simulink model "Soundtest"  (R2021a)
settings: Solver=FixedStepAuto  StartTime=0.0  StopTime=90  RelTol=1e-3
undefined symbols (not defined in the file): fdesignblkfcn, gcbh
libraries: simulink x25, simulink_extras x14, hdlsllib x9, eeGeneralControl x5, dspvision x4, commrandsrc3 x4, commutil2 x1
(part 1 of 5)
settings Model: Creator=PS  LastModifiedBy=PS

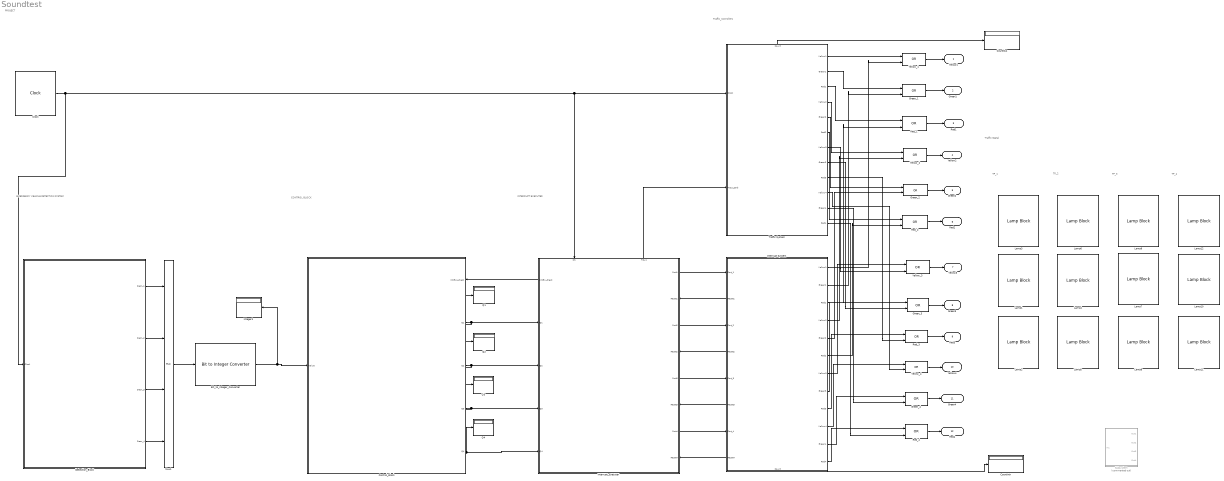
== system Soundtest ==
  note: INTERRUPT EXECUTER
  note: PROJECT
  note: CONTROL BLOCK
  note: EMERGENCY VEHICLE
      | 												DETECTION SYSTEM
  note: Traffic Signal
  note: Traffic_Conrollers
  note: TP_3
  note: TP_4
  note: TP_2
  note: TP_1
  " Control_Block" : Subsystem
      settings: PortSchema="{\"entries\":[{\"content\":{\"sides\":[{\"content\":{\"connectorIds\":[\"In1\"]},\"type\":\"ConnectorPlacement.EquallySpacedRectSide\",\"uuid\":\"7bdef495-49f6-4a33-afc1-3adee0384943\"},{\"content\":{\"connectorIds\":[\"In2\",\"Out1\",\"Out2\",\"Out3\",\"Out4\"],\"side\":\"RIGHT\"},\"type\":\"ConnectorPlacement.EquallySpacedRectSide\",\"uuid\":\"f7d0219f-f955-47d8-95dc-bc644c2b66ac\"},{\"content\":{\"connectorIds\":[],\"side\":\"TOP\"},\"type\":\"ConnectorPlacement.EquallySpacedRectSide\",\"uuid\":\"78ec8059-9416-4ba2-a7c7-38e9e6d506d5\"}]},\"type\":\"ConnectorPlacement.EquallySpacedConnector\",\"uuid\":\"6f2568f4-98e0-4465-825d-49049fff1cf4\"}],\"packageUris\":[\"http://schema.mathworks.com/mf0/Connector/R2020b\"],\"version\":\"1.0\"}"
  Bit_to_Integer_Converter : commutil2/Bit to Integer Converter  nbits=4  bitOrder=LSB first  signedOutputValues=Unsigned  outDtype=Inherit via internal rule  outDtypeSigned=Inherit via internal rule
  Clock : simulink_extras/Flip Flops/Clock  period=2
  CountIntr : Display
  CountSys : Display
  Detection_Block : Subsystem
  Green_{1..4} (4 alike) : Logic  Operator=OR  IconShape=distinctive  AllPortsSameDT=off  OutDataTypeStr=boolean
  Integer1 : Display
  Interrupt System : Subsystem
      settings: PortSchema="{\"entries\":[{\"content\":{\"sides\":[{\"content\":{\"connectorIds\":[\"In1\",\"Out14\",\"In2\",\"Out15\",\"In3\",\"Out16\",\"In4\",\"Out17\"]},\"type\":\"ConnectorPlacement.EquallySpacedRectSide\",\"uuid\":\"dd9361c9-50ac-49b9-98e3-b3d02327774e\"},{\"content\":{\"connectorIds\":[\"Out1\",\"Out2\",\"Out3\",\"Out4\",\"Out5\",\"Out6\",\"Out7\",\"Out8\",\"Out9\",\"Out10\",\"Out11\",\"Out12\"],\"side\":\"RIGHT\"},\"type\":\"ConnectorPlacement.EquallySpacedRectSide\",\"uuid\":\"f7e4faee-0171-4d20-8361-b22acdf13a20\"},{\"content\":{\"connectorIds\":[],\"side\":\"TOP\"},\"type\":\"ConnectorPlacement.EquallySpacedRectSide\",\"uuid\":\"5413f0d1-8ff5-4455-b45d-8db19df6353c\"},{\"content\":{\"connectorIds\":[\"Out13\"],\"side\":\"BOTTOM\"},\"type\":\"ConnectorPlacement.EquallySpacedRectSide\",\"uuid\":\"93b26c12-c259-4f39-b0b9-3af84b79bd60\"}]},\"type\":\"ConnectorPlacement.EquallySpacedConnector\",\"uuid\":\"eebdce44-6a00-4600-b51a-a6b58439fb08\"}],\"packageUris\":[\"http://schema.mathworks.com/mf0/Connector/R2020b\"],\"version\":\"1.0\"}"
  Interrupt_Executer : Subsystem
      settings: PortSchema="{\"entries\":[{\"content\":{\"sides\":[{\"content\":{\"connectorIds\":[\"Out6\",\"In1\",\"In2\",\"In3\",\"In4\"]},\"type\":\"ConnectorPlacement.EquallySpacedRectSide\",\"uuid\":\"f4bdf6e7-e5e7-43ea-b16b-e41e60f72b46\"},{\"content\":{\"connectorIds\":[\"Out1\",\"In6\",\"Out2\",\"In7\",\"Out3\",\"In8\",\"Out4\",\"In9\"],\"side\":\"RIGHT\"},\"type\":\"ConnectorPlacement.EquallySpacedRectSide\",\"uuid\":\"e5b218e6-0b4a-46b0-9989-01396b28dd8c\"},{\"content\":{\"connectorIds\":[\"In5\",\"Out5\"],\"side\":\"TOP\"},\"type\":\"ConnectorPlacement.EquallySpacedRectSide\",\"uuid\":\"ea6d06c9-d4c6-4cbd-a699-b09547b6713d\"}]},\"type\":\"ConnectorPlacement.EquallySpacedConnector\",\"uuid\":\"db6fa2d9-b0de-4c1a-aad1-7814046e63dd\"}],\"packageUris\":[\"http://schema.mathworks.com/mf0/Connector/R2020b\"],\"version\":\"1.0\"}"
  Lamp{1..12} (12 alike) : LampBlock
  Mux1 : Mux
  Q{1..4} (4 alike) : Display
  Red_{1..4} (4 alike) : Logic  Operator=OR  IconShape=distinctive  AllPortsSameDT=off  OutDataTypeStr=boolean
  Subsystem : Subsystem  Commented=on
  Traffic System : Subsystem
      settings: PortSchema="{\"entries\":[{\"content\":{\"sides\":[{\"content\":{\"connectorIds\":[\"In1\",\"In2\"]},\"type\":\"ConnectorPlacement.EquallySpacedRectSide\",\"uuid\":\"23d8ab70-c3d3-4b79-b104-f032a6dab7cf\"},{\"content\":{\"connectorIds\":[\"Out1\",\"Out2\",\"Out3\",\"Out4\",\"Out5\",\"Out6\",\"Out7\",\"Out8\",\"Out9\",\"Out10\",\"Out11\",\"Out12\"],\"side\":\"RIGHT\"},\"type\":\"ConnectorPlacement.EquallySpacedRectSide\",\"uuid\":\"7588026f-a2a4-4010-ad00-9eb40a03c993\"},{\"content\":{\"connectorIds\":[\"Out13\"],\"side\":\"TOP\"},\"type\":\"ConnectorPlacement.EquallySpacedRectSide\",\"uuid\":\"55eb16ed-4094-4229-af86-8dde9acd4f47\"}]},\"type\":\"ConnectorPlacement.EquallySpacedConnector\",\"uuid\":\"d987693c-4e87-4150-befb-2339b1a44195\"}],\"packageUris\":[\"http://schema.mathworks.com/mf0/Connector/R2020b\"],\"version\":\"1.0\"}"
  Yellow_{1..4} (4 alike) : Logic  Operator=OR  IconShape=distinctive  AllPortsSameDT=off  OutDataTypeStr=boolean
  Yellow1 : Outport  VectorParamsAs1DForOutWhenUnconnected=off
  Green1 : Outport  Port=2  VectorParamsAs1DForOutWhenUnconnected=off
  Red1 : Outport  Port=3  VectorParamsAs1DForOutWhenUnconnected=off
  Yellow2 : Outport  Port=4  VectorParamsAs1DForOutWhenUnconnected=off
  Green2 : Outport  Port=5  VectorParamsAs1DForOutWhenUnconnected=off
  Red2 : Outport  Port=6  VectorParamsAs1DForOutWhenUnconnected=off
  Yellow3 : Outport  Port=7  VectorParamsAs1DForOutWhenUnconnected=off
  Green3 : Outport  Port=8  VectorParamsAs1DForOutWhenUnconnected=off
  Red3 : Outport  Port=9  VectorParamsAs1DForOutWhenUnconnected=off
  Yellow4 : Outport  Port=10  VectorParamsAs1DForOutWhenUnconnected=off
  Green4 : Outport  Port=11  VectorParamsAs1DForOutWhenUnconnected=off
  Red4 : Outport  Port=12  VectorParamsAs1DForOutWhenUnconnected=off
  wires:
  Yellow_1/1 -> Yellow1/1
  Traffic System/1(Yellow1) -> Yellow_1/1
  Interrupt System/1(Yellow1) -> Yellow_1/2
  Traffic System/2(Green1) -> Green_1/1
  Interrupt System/2(Green1) -> Green_1/2
  Traffic System/3(Red1) -> Red_1/1
  Interrupt System/3(Red1) -> Red_1/2
  Traffic System/4(Yellow2) -> Yellow_2/1
  Interrupt System/4(Yellow2) -> Yellow_2/2
  Traffic System/5(Green2) -> Green_2/1
  Interrupt System/5(Green2) -> Green_2/2
  Green_1/1 -> Green1/1
  Red_1/1 -> Red1/1
  Yellow_2/1 -> Yellow2/1
  Green_2/1 -> Green2/1
  Traffic System/6(Red2) -> Red_2/1
  Interrupt System/6(Red2) -> Red_2/2
  Interrupt System/7(Yellow3) -> Yellow_3/1
  Traffic System/7(Yellow3) -> Yellow_3/2
  Traffic System/8(Green3) -> Green_3/2
  Interrupt System/8(Green3) -> Green_3/1
  Interrupt System/9(Red3) -> Red_3/1
  Traffic System/9(Red3) -> Red_3/2
  Interrupt System/10(Yellow4) -> Yellow_4/1
  Traffic System/10(Yellow4) -> Yellow_4/2
  Traffic System/11(Green4) -> Green_4/2
  Interrupt System/11(Green4) -> Green_4/1
  Interrupt System/12(Red4) -> Red_4/1
  Traffic System/12(Red4) -> Red_4/2
  Red_4/1 -> Red4/1
  Green_4/1 -> Green4/1
  Yellow_4/1 -> Yellow4/1
  Red_3/1 -> Red3/1
  Green_3/1 -> Green3/1
  Red_2/1 -> Red2/1
  Yellow_3/1 -> Yellow3/1
  Bit_to_Integer_Converter/1 -> Integer1/1, " Control_Block"/1(Value)
  Mux1/1 -> Bit_to_Integer_Converter/1
  Interrupt System/14(Reset1) -> Interrupt_Executer/6(Reset1)
  Interrupt System/15(Reset2) -> Interrupt_Executer/7(Reset2)
  Interrupt System/16(Reset3) -> Interrupt_Executer/8(Reset3)
  Interrupt System/17(Reset4) -> Interrupt_Executer/9(Reset4)
  Interrupt_Executer/5(TrSys) -> Traffic System/2(TrSys_Enb)
  Interrupt_Executer/6(IntrEx_check) -> " Control_Block"/2(IntrExc_check)
  Interrupt_Executer/1(Port1) -> Interrupt System/1(Port_1)
  Interrupt_Executer/2(Port2) -> Interrupt System/2(Port_2)
  Interrupt_Executer/3(Port3) -> Interrupt System/3(Port_3)
  Interrupt_Executer/4(Port4) -> Interrupt System/4(Port_4)
  " Control_Block"/1(Q1) -> Q1/1, Interrupt_Executer/1(Q1)
  " Control_Block"/2(Q2) -> Q2/1, Interrupt_Executer/2(Q2)
  " Control_Block"/3(Q3) -> Q3/1, Interrupt_Executer/3(Q3)
  " Control_Block"/4(Q4) -> Q4/1, Interrupt_Executer/4(Q4)
  Interrupt System/13(Count) -> CountIntr/1
  Traffic System/13(Count) -> CountSys/1
  Detection_Block/1(Decn_1) -> Mux1/1
  Detection_Block/2(Decn_2) -> Mux1/2
  Detection_Block/3(Decn_3) -> Mux1/3
  Detection_Block/4(Decn_4) -> Mux1/4
  Clock/1 -> Detection_Block/1(Clock), Traffic System/1(Clock), Interrupt_Executer/5(Clk)

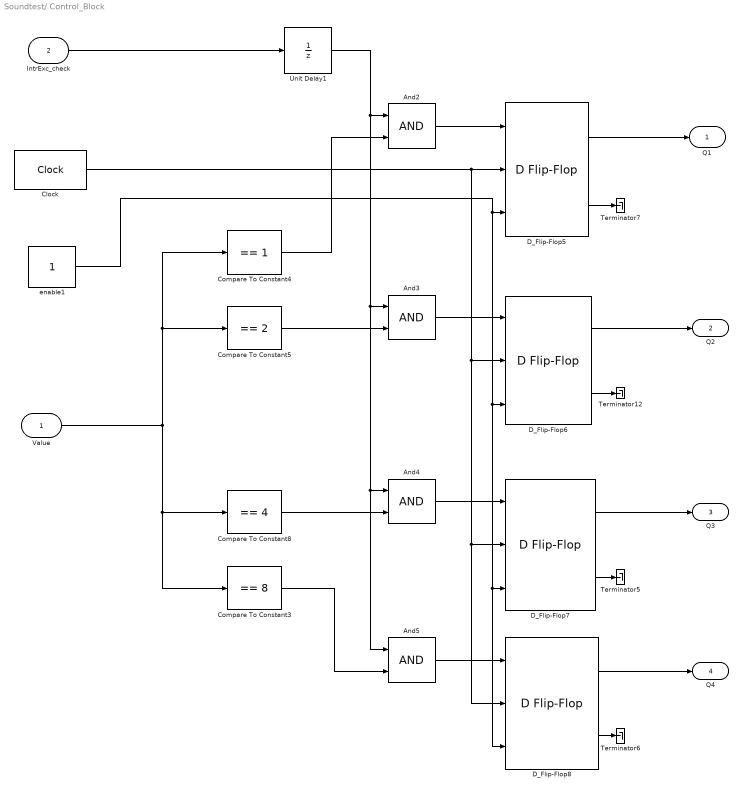
== system Soundtest/ Control_Block ==
  Value : Inport
  IntrExc_check : Inport  Port=2
  And{2..5} (4 alike) : Logic  IconShape=distinctive  AllPortsSameDT=off  OutDataTypeStr=boolean
  Clock : simulink_extras/Flip Flops/Clock  period=4
  Compare To Constant3 : simulink/Logic and Bit Operations/Compare To Constant  relop===  const=8  OutDataTypeStr=boolean
  Compare To Constant4 : simulink/Logic and Bit Operations/Compare To Constant  relop===  const=1  OutDataTypeStr=boolean
  Compare To Constant5 : simulink/Logic and Bit Operations/Compare To Constant  relop===  const=2  OutDataTypeStr=boolean
  Compare To Constant8 : simulink/Logic and Bit Operations/Compare To Constant  relop===  const=4  OutDataTypeStr=boolean
  D_Flip-Flop{5..8} (4 alike) : simulink_extras/Flip Flops/D Flip-Flop
  Terminator{5..7,12} (4 alike) : Terminator
  Unit Delay1 : UnitDelay  SampleTime=-1  HasFrameUpgradeWarning=on
  enable1 : Constant  OutDataTypeStr=boolean
  Q1 : Outport
  Q2 : Outport  Port=2
  Q3 : Outport  Port=3
  Q4 : Outport  Port=4
  wires:
  D_Flip-Flop8/1 -> Q4/1
  D_Flip-Flop5/1 -> Q1/1
  Clock/1 -> D_Flip-Flop5/2, D_Flip-Flop6/2, D_Flip-Flop7/2, D_Flip-Flop8/2
  enable1/1 -> D_Flip-Flop8/3, D_Flip-Flop7/3, D_Flip-Flop6/3, D_Flip-Flop5/3
  Compare To Constant5/1 -> And3/2
  Value/1 -> Compare To Constant4/1, Compare To Constant5/1, Compare To Constant3/1, Compare To Constant8/1
  And4/1 -> D_Flip-Flop7/1
  D_Flip-Flop6/2 -> Terminator12/1
  D_Flip-Flop6/1 -> Q2/1
  D_Flip-Flop7/1 -> Q3/1
  Compare To Constant8/1 -> And4/2
  D_Flip-Flop7/2 -> Terminator5/1
  D_Flip-Flop5/2 -> Terminator7/1
  And3/1 -> D_Flip-Flop6/1
  Unit Delay1/1 -> And2/1, And5/1, And4/1, And3/1
  Compare To Constant3/1 -> And5/2
  D_Flip-Flop8/2 -> Terminator6/1
  Compare To Constant4/1 -> And2/2
  And2/1 -> D_Flip-Flop5/1
  And5/1 -> D_Flip-Flop8/1
  IntrExc_check/1 -> Unit Delay1/1

== system Soundtest/Detection_Block ==
  Clock : Inport
  AND_{1..4} (4 alike) : Logic  IconShape=distinctive  AllPortsSameDT=off  OutDataTypeStr=boolean
  Ambulance_Detectors : Subsystem
  Constant : Constant  OutDataTypeStr=boolean
  D Flip-Flop1 : simulink_extras/Flip Flops/D Flip-Flop
  Enable : Constant  OutDataTypeStr=boolean
  Input_Sensors : Subsystem
  Scope : Scope  NumInputPorts=3
  Terminator2 : Terminator
  Decn_1 : Outport
  Decn_2 : Outport  Port=2
  Decn_3 : Outport  Port=3
  Decn_4 : Outport  Port=4
  wires:
  Input_Sensors/1(Inp_1) -> Ambulance_Detectors/1(Inp_1)
  Ambulance_Detectors/1(Filter_Out) -> Scope/1
  Input_Sensors/3(Inp_3) -> Ambulance_Detectors/3(Inp_3)
  Ambulance_Detectors/2(Mag_Out) -> Scope/2
  Input_Sensors/2(Inp_2) -> Ambulance_Detectors/2(Inp_2)
  Input_Sensors/4(Inp_4) -> Ambulance_Detectors/4(Inp_4)
  Ambulance_Detectors/3(Decn_1) -> AND_1/1, Scope/3
  Ambulance_Detectors/4(Decn_2) -> AND_2/1
  Constant/1 -> D Flip-Flop1/1
  D Flip-Flop1/2 -> Terminator2/1
  Enable/1 -> D Flip-Flop1/3
  Clock/1 -> D Flip-Flop1/2
  AND_2/1 -> Decn_2/1
  AND_3/1 -> Decn_3/1
  Ambulance_Detectors/5(Decn_3) -> AND_3/1
  Ambulance_Detectors/6(Decn_4) -> AND_4/1
  AND_4/1 -> Decn_4/1
  D Flip-Flop1/1 -> AND_1/2, AND_2/2, AND_3/2, AND_4/2
  AND_1/1 -> Decn_1/1

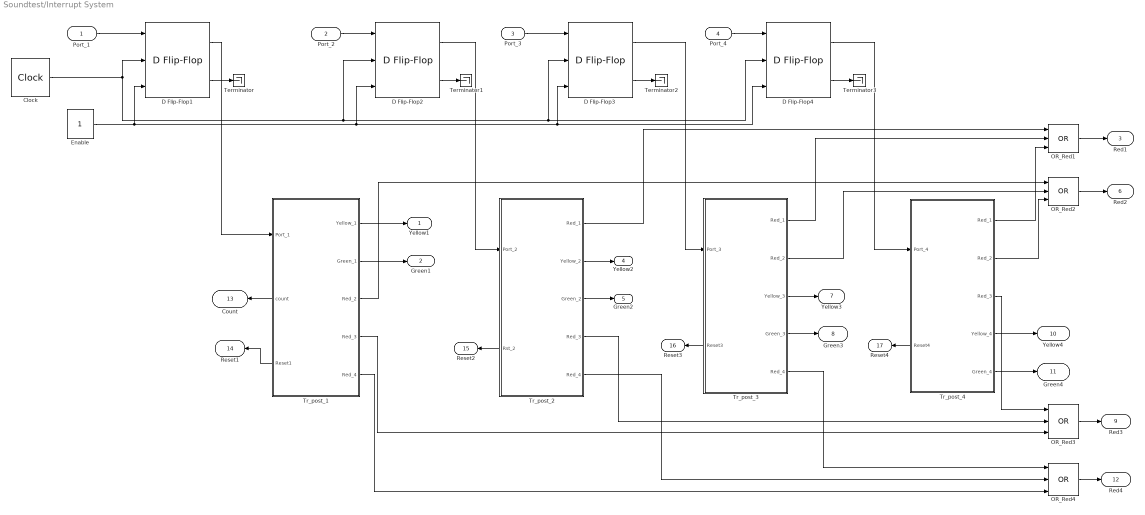
== system Soundtest/Interrupt System ==
  Port_1 : Inport
  Port_2 : Inport  Port=2
  Port_3 : Inport  Port=3
  Port_4 : Inport  Port=4
  Clock : simulink_extras/Flip Flops/Clock  period=2
  D Flip-Flop{1..4} (4 alike) : simulink_extras/Flip Flops/D Flip-Flop
  Enable : Constant  OutDataTypeStr=boolean
  OR_Red{1..4} (4 alike) : Logic  Operator=OR  Inputs=3  IconShape=distinctive  AllPortsSameDT=off  OutDataTypeStr=boolean
  Terminator{,1..3} (4 alike) : Terminator
  Tr_post_1 : Subsystem
      settings: PortSchema="{\"entries\":[{\"content\":{\"sides\":[{\"content\":{\"connectorIds\":[\"In1\",\"Out6\",\"Out7\"]},\"type\":\"ConnectorPlacement.EquallySpacedRectSide\",\"uuid\":\"ab8f469e-3332-475a-83d5-afbd6f66f4e6\"},{\"content\":{\"connectorIds\":[\"Out1\",\"Out2\",\"Out3\",\"Out4\",\"Out5\"],\"side\":\"RIGHT\"},\"type\":\"ConnectorPlacement.EquallySpacedRectSide\",\"uuid\":\"6823faed-dca4-4af2-a519-b6f8f71579c8\"},{\"content\":{\"connectorIds\":[],\"side\":\"TOP\"},\"type\":\"ConnectorPlacement.EquallySpacedRectSide\",\"uuid\":\"8d9facd3-edb6-42bc-be5d-0022a243b86f\"}]},\"type\":\"ConnectorPlacement.EquallySpacedConnector\",\"uuid\":\"a2e4fdf2-469e-412a-bc2f-0a5c51d0db72\"}],\"packageUris\":[\"http://schema.mathworks.com/mf0/Connector/R2020b\"],\"version\":\"1.0\"}"
  Tr_post_2 : Subsystem
      settings: PortSchema="{\"entries\":[{\"content\":{\"sides\":[{\"content\":{\"connectorIds\":[\"In1\",\"Out6\"]},\"type\":\"ConnectorPlacement.EquallySpacedRectSide\",\"uuid\":\"cf8efb98-dcb3-4b52-bb29-44068cf36b42\"},{\"content\":{\"connectorIds\":[\"Out1\",\"Out2\",\"Out3\",\"Out4\",\"Out5\"],\"side\":\"RIGHT\"},\"type\":\"ConnectorPlacement.EquallySpacedRectSide\",\"uuid\":\"3b505268-83a1-4950-b579-e5c30ad50a49\"},{\"content\":{\"connectorIds\":[],\"side\":\"TOP\"},\"type\":\"ConnectorPlacement.EquallySpacedRectSide\",\"uuid\":\"d6f0b650-deb9-4fd5-a2d1-5d40893a956e\"}]},\"type\":\"ConnectorPlacement.EquallySpacedConnector\",\"uuid\":\"7382f276-3b35-4664-8acb-0fe9e679eb95\"}],\"packageUris\":[\"http://schema.mathworks.com/mf0/Connector/R2020b\"],\"version\":\"1.0\"}"
  Tr_post_3 : Subsystem
      settings: PortSchema="{\"entries\":[{\"content\":{\"sides\":[{\"content\":{\"connectorIds\":[\"In1\",\"Out6\"]},\"type\":\"ConnectorPlacement.EquallySpacedRectSide\",\"uuid\":\"cf8efb98-dcb3-4b52-bb29-44068cf36b42\"},{\"content\":{\"connectorIds\":[\"Out1\",\"Out2\",\"Out3\",\"Out4\",\"Out5\"],\"side\":\"RIGHT\"},\"type\":\"ConnectorPlacement.EquallySpacedRectSide\",\"uuid\":\"3b505268-83a1-4950-b579-e5c30ad50a49\"},{\"content\":{\"connectorIds\":[],\"side\":\"TOP\"},\"type\":\"ConnectorPlacement.EquallySpacedRectSide\",\"uuid\":\"d6f0b650-deb9-4fd5-a2d1-5d40893a956e\"}]},\"type\":\"ConnectorPlacement.EquallySpacedConnector\",\"uuid\":\"7382f276-3b35-4664-8acb-0fe9e679eb95\"}],\"packageUris\":[\"http://schema.mathworks.com/mf0/Connector/R2020b\"],\"version\":\"1.0\"}"
  Tr_post_4 : Subsystem
      settings: PortSchema="{\"entries\":[{\"content\":{\"sides\":[{\"content\":{\"connectorIds\":[\"In1\",\"Out6\"]},\"type\":\"ConnectorPlacement.EquallySpacedRectSide\",\"uuid\":\"cf8efb98-dcb3-4b52-bb29-44068cf36b42\"},{\"content\":{\"connectorIds\":[\"Out1\",\"Out2\",\"Out3\",\"Out4\",\"Out5\"],\"side\":\"RIGHT\"},\"type\":\"ConnectorPlacement.EquallySpacedRectSide\",\"uuid\":\"3b505268-83a1-4950-b579-e5c30ad50a49\"},{\"content\":{\"connectorIds\":[],\"side\":\"TOP\"},\"type\":\"ConnectorPlacement.EquallySpacedRectSide\",\"uuid\":\"d6f0b650-deb9-4fd5-a2d1-5d40893a956e\"}]},\"type\":\"ConnectorPlacement.EquallySpacedConnector\",\"uuid\":\"7382f276-3b35-4664-8acb-0fe9e679eb95\"}],\"packageUris\":[\"http://schema.mathworks.com/mf0/Connector/R2020b\"],\"version\":\"1.0\"}"
  Yellow1 : Outport
  Green1 : Outport  Port=2
  Red1 : Outport  Port=3
  Yellow2 : Outport  Port=4
  Green2 : Outport  Port=5
  Red2 : Outport  Port=6
  Yellow3 : Outport  Port=7
  Green3 : Outport  Port=8
  Red3 : Outport  Port=9
  Yellow4 : Outport  Port=10
  Green4 : Outport  Port=11
  Red4 : Outport  Port=12
  Count : Outport  Port=13
  Reset1 : Outport  Port=14
  Reset2 : Outport  Port=15
  Reset3 : Outport  Port=16
  Reset4 : Outport  Port=17
  wires:
  Tr_post_2/2(Yellow_2) -> Yellow2/1
  Tr_post_3/3(Yellow_3) -> Yellow3/1
  Tr_post_3/4(Green_3) -> Green3/1
  Tr_post_4/5(Green_4) -> Green4/1
  Tr_post_4/4(Yellow_4) -> Yellow4/1
  Tr_post_2/3(Green_2) -> Green2/1
  OR_Red1/1 -> Red1/1
  Tr_post_1/2(Green_1) -> Green1/1
  Tr_post_1/1(Yellow_1) -> Yellow1/1
  OR_Red2/1 -> Red2/1
  OR_Red4/1 -> Red4/1
  OR_Red3/1 -> Red3/1
  Tr_post_2/1(Red_1) -> OR_Red1/1
  Tr_post_3/1(Red_1) -> OR_Red1/2
  Tr_post_4/1(Red_1) -> OR_Red1/3
  Tr_post_1/3(Red_2) -> OR_Red2/1
  Tr_post_3/2(Red_2) -> OR_Red2/2
  Tr_post_4/2(Red_2) -> OR_Red2/3
  Tr_post_1/4(Red_3) -> OR_Red3/3
  Tr_post_2/4(Red_3) -> OR_Red3/2
  Tr_post_4/3(Red_3) -> OR_Red3/1
  Tr_post_1/5(Red_4) -> OR_Red4/3
  Tr_post_2/5(Red_4) -> OR_Red4/2
  Tr_post_3/5(Red_4) -> OR_Red4/1
  Tr_post_1/7(Reset1) -> Reset1/1
  Tr_post_2/6(Rst_2) -> Reset2/1
  Tr_post_3/6(Reset3) -> Reset3/1
  Tr_post_4/6(Reset4) -> Reset4/1
  D Flip-Flop1/1 -> Tr_post_1/1(Port_1)
  Port_1/1 -> D Flip-Flop1/1
  D Flip-Flop1/2 -> Terminator/1
  D Flip-Flop2/1 -> Tr_post_2/1(Port_2)
  D Flip-Flop2/2 -> Terminator1/1
  Port_2/1 -> D Flip-Flop2/1
  D Flip-Flop3/1 -> Tr_post_3/1(Port_3)
  Port_3/1 -> D Flip-Flop3/1
  D Flip-Flop3/2 -> Terminator2/1
  Port_4/1 -> D Flip-Flop4/1
  D Flip-Flop4/2 -> Terminator3/1
  Clock/1 -> D Flip-Flop1/2, D Flip-Flop2/2, D Flip-Flop4/2, D Flip-Flop3/2
  Enable/1 -> D Flip-Flop4/3, D Flip-Flop3/3, D Flip-Flop2/3, D Flip-Flop1/3
  D Flip-Flop4/1 -> Tr_post_4/1(Port_4)
  Tr_post_1/6(count) -> Count/1

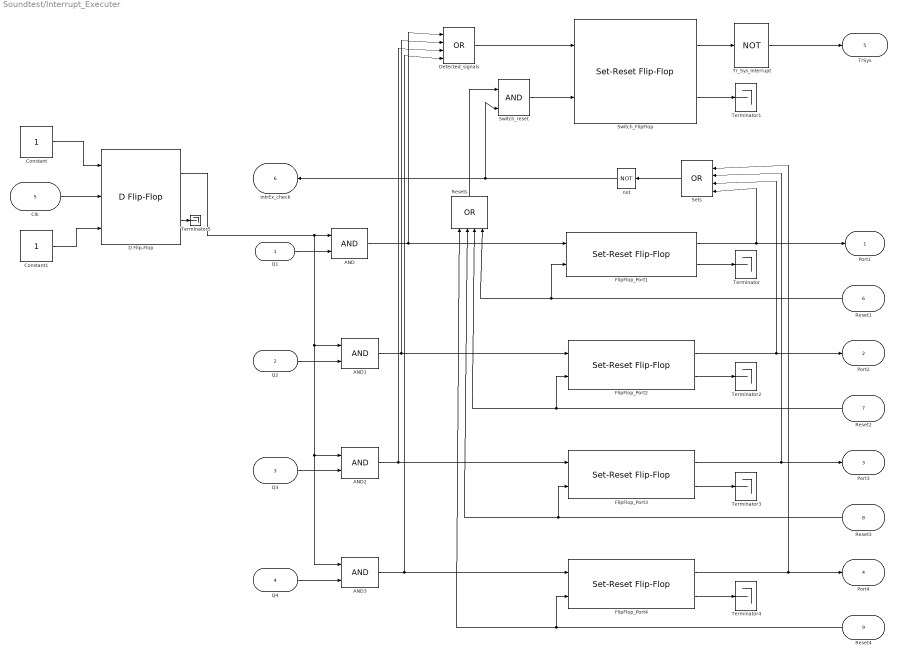
== system Soundtest/Interrupt_Executer ==
  Q1 : Inport
  Q2 : Inport  Port=2
  Q3 : Inport  Port=3
  Q4 : Inport  Port=4
  Clk : Inport  Port=5
  Reset1 : Inport  Port=6
  Reset2 : Inport  Port=7
  Reset3 : Inport  Port=8
  Reset4 : Inport  Port=9
  AND{,1..3} (4 alike) : Logic  IconShape=distinctive  AllPortsSameDT=off  OutDataTypeStr=boolean
  Constant : Constant  OutDataTypeStr=boolean
  Constant1 : Constant  OutDataTypeStr=boolean
  D Flip-Flop : simulink_extras/Flip Flops/D Flip-Flop
  Detected_signals : Logic  Operator=OR  Inputs=4  IconShape=distinctive  AllPortsSameDT=off  OutDataTypeStr=boolean
  FlipFlop_Port{1..4} (4 alike) : eeGeneralControl/Set-Reset Flip-Flop  LabelModeActiveChoice=Discrete  UndefState=Set  Q0=0  Ts=-1
      settings: SourceProductBaseCode=PS
  Resets : Logic  Operator=OR  Inputs=4  IconShape=distinctive  AllPortsSameDT=off  OutDataTypeStr=boolean
  Sets : Logic  Operator=OR  Inputs=4  IconShape=distinctive  AllPortsSameDT=off  OutDataTypeStr=boolean
  Switch_FlipFlop : eeGeneralControl/Set-Reset Flip-Flop  LabelModeActiveChoice=Discrete  UndefState=Set  Q0=0  Ts=-1
      settings: SourceProductBaseCode=PS
  Switch_reset : Logic  IconShape=distinctive  AllPortsSameDT=off  OutDataTypeStr=boolean
  Terminator{,1..5} (6 alike) : Terminator
  Tr_Sys_Interrupt : Logic  Operator=NOT  Inputs=4  IconShape=distinctive  AllPortsSameDT=off  OutDataTypeStr=boolean
  not : Logic  Operator=NOT  Inputs=4  IconShape=distinctive  AllPortsSameDT=off  OutDataTypeStr=boolean
  Port1 : Outport
  Port2 : Outport  Port=2
  Port3 : Outport  Port=3
  Port4 : Outport  Port=4
  TrSys : Outport  Port=5
  IntrEx_check : Outport  Port=6
  wires:
  FlipFlop_Port1/1 -> Sets/4, Port1/1
  Switch_reset/1 -> Switch_FlipFlop/2
  Reset2/1 -> FlipFlop_Port2/2, Resets/3
  FlipFlop_Port2/2 -> Terminator2/1
  Switch_FlipFlop/1 -> Tr_Sys_Interrupt/1
  FlipFlop_Port2/1 -> Sets/3, Port2/1
  AND1/1 -> Detected_signals/2, FlipFlop_Port2/1
  AND3/1 -> Detected_signals/4, FlipFlop_Port4/1
  Reset3/1 -> FlipFlop_Port3/2, Resets/2
  Switch_FlipFlop/2 -> Terminator1/1
  not/1 -> Switch_reset/2, IntrEx_check/1
  Reset1/1 -> Resets/4, FlipFlop_Port1/2
  Sets/1 -> not/1
  Resets/1 -> Switch_reset/1
  FlipFlop_Port3/2 -> Terminator3/1
  AND2/1 -> Detected_signals/3, FlipFlop_Port3/1
  FlipFlop_Port3/1 -> Sets/2, Port3/1
  Tr_Sys_Interrupt/1 -> TrSys/1
  FlipFlop_Port4/2 -> Terminator4/1
  Reset4/1 -> FlipFlop_Port4/2, Resets/1
  Detected_signals/1 -> Switch_FlipFlop/1
  FlipFlop_Port4/1 -> Sets/1, Port4/1
  FlipFlop_Port1/2 -> Terminator/1
  AND/1 -> Detected_signals/1, FlipFlop_Port1/1
  Constant/1 -> D Flip-Flop/1
  Clk/1 -> D Flip-Flop/2
  Constant1/1 -> D Flip-Flop/3
  Q1/1 -> AND/2
  D Flip-Flop/1 -> AND3/1, AND2/1, AND1/1, AND/1
  Q2/1 -> AND1/2
  Q3/1 -> AND2/2
  Q4/1 -> AND3/2
  D Flip-Flop/2 -> Terminator5/1

== system Soundtest/Subsystem ==
  note: Binary_Generator
  In1 : Inport
  AND{,1..3} (4 alike) : Logic  IconShape=distinctive  AllPortsSameDT=off  OutDataTypeStr=boolean
  Bernoulli Binary Generator : commrandsrc3/Bernoulli Binary Generator  ProbabilityOfZero=1  SeedSource=Auto  Seed=0  SampleTime=1  SamplesPerFrame=1  OutputDataType=boolean  SimulateUsing=Interpreted execution
  Bernoulli Binary Generator1 : commrandsrc3/Bernoulli Binary Generator  ProbabilityOfZero=0.8  SeedSource=Auto  Seed=0  SampleTime=1  SamplesPerFrame=1  OutputDataType=boolean  SimulateUsing=Interpreted execution
  Bernoulli Binary Generator2 : commrandsrc3/Bernoulli Binary Generator  ProbabilityOfZero=0.8  SeedSource=Auto  Seed=0  SampleTime=1  SamplesPerFrame=1  OutputDataType=boolean  SimulateUsing=Interpreted execution
  Bernoulli Binary Generator3 : commrandsrc3/Bernoulli Binary Generator  ProbabilityOfZero=0.8  SeedSource=Auto  Seed=0  SampleTime=1  SamplesPerFrame=1  OutputDataType=boolean  SimulateUsing=Interpreted execution
  Out1 : Outport
  Out2 : Outport  Port=2
  Out3 : Outport  Port=3
  Out4 : Outport  Port=4
  wires:
  Bernoulli Binary Generator/1 -> AND/1
  Bernoulli Binary Generator3/1 -> AND3/1
  Bernoulli Binary Generator2/1 -> AND2/1
  Bernoulli Binary Generator1/1 -> AND1/2
  In1/1 -> AND3/2, AND2/2, AND1/1, AND/2
  AND2/1 -> Out3/1
  AND3/1 -> Out4/1
  AND1/1 -> Out2/1
  AND/1 -> Out1/1

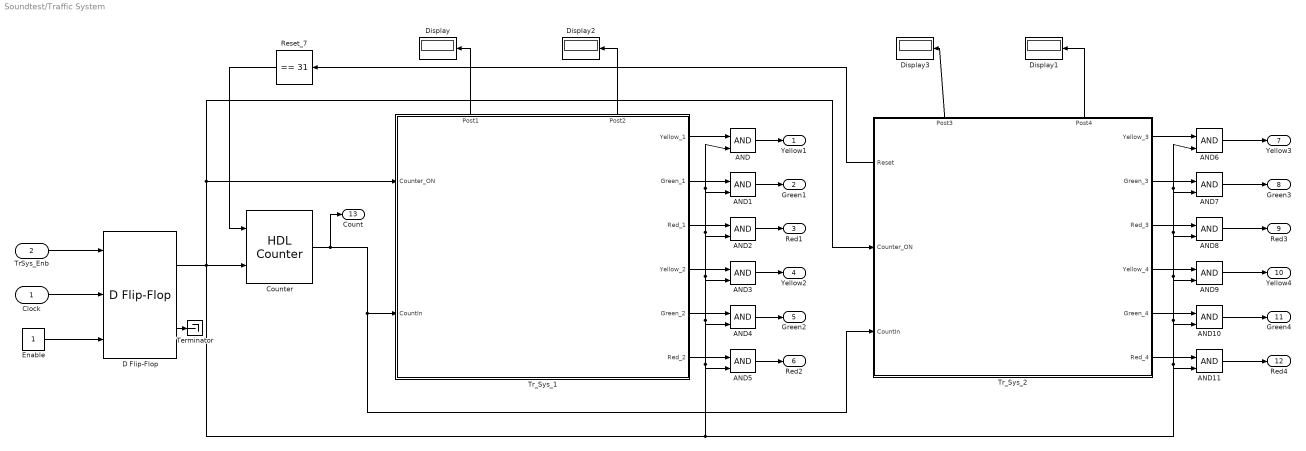
== system Soundtest/Traffic System ==
  Clock : Inport
  TrSys_Enb : Inport  Port=2
  AND{,1..11} (12 alike) : Logic  IconShape=distinctive  AllPortsSameDT=off  OutDataTypeStr=boolean
  Counter : hdlsllib/Sources/HDL Counter  CountType=Count limited  CountInit=0  CountStep=1  CountMax=31  CountFromType=Initial value  CountFrom=0  CountResetPort=on  CountLoadPort=off  CountEnbPort=on  CountDirPort=off  CountHitOutputPort=off  CountDataType=Unsigned  CountWordLen=8  CountFracLen=0  CountSampTime=1
  D Flip-Flop : simulink_extras/Flip Flops/D Flip-Flop
  Display{,1..3} (4 alike) : Display
  Enable : Constant  OutDataTypeStr=boolean
  Reset_7 : simulink/Logic and Bit Operations/Compare To Constant  relop===  const=31  OutDataTypeStr=boolean
  Terminator : Terminator
  Tr_Sys_1 : Subsystem
      settings: PortSchema="{\"entries\":[{\"content\":{\"sides\":[{\"content\":{\"connectorIds\":[\"In1\",\"In2\"]},\"type\":\"ConnectorPlacement.EquallySpacedRectSide\",\"uuid\":\"cd6a573a-f63a-4267-a232-9eb42b0e4457\"},{\"content\":{\"connectorIds\":[\"Out1\",\"Out2\",\"Out3\",\"Out4\",\"Out5\",\"Out6\"],\"side\":\"RIGHT\"},\"type\":\"ConnectorPlacement.EquallySpacedRectSide\",\"uuid\":\"f6eb4910-c6df-488e-ab3b-2d26710c7ea4\"},{\"content\":{\"connectorIds\":[\"Out7\",\"Out8\"],\"side\":\"TOP\"},\"type\":\"ConnectorPlacement.EquallySpacedRectSide\",\"uuid\":\"a673d499-f1f0-4298-be23-50c47df79d07\"}]},\"type\":\"ConnectorPlacement.EquallySpacedConnector\",\"uuid\":\"fa6e7a6f-15f6-4fb6-9f68-54e163a559b7\"}],\"packageUris\":[\"http://schema.mathworks.com/mf0/Connector/R2020b\"],\"version\":\"1.0\"}"
  Tr_Sys_2 : Subsystem
      settings: PortSchema="{\"entries\":[{\"content\":{\"sides\":[{\"content\":{\"connectorIds\":[\"Out9\",\"In1\",\"In2\"]},\"type\":\"ConnectorPlacement.EquallySpacedRectSide\",\"uuid\":\"f688e7f2-a4b0-4876-aa54-3ea0bbaacfd9\"},{\"content\":{\"connectorIds\":[\"Out1\",\"Out2\",\"Out3\",\"Out4\",\"Out5\",\"Out6\"],\"side\":\"RIGHT\"},\"type\":\"ConnectorPlacement.EquallySpacedRectSide\",\"uuid\":\"7fe066cd-bdaf-47f1-a6ea-f29d6eb723dd\"},{\"content\":{\"connectorIds\":[\"Out7\",\"Out8\"],\"side\":\"TOP\"},\"type\":\"ConnectorPlacement.EquallySpacedRectSide\",\"uuid\":\"39c29f91-5efa-4dbe-99ee-6bedb48eb38c\"},{\"content\":{\"connectorIds\":[],\"side\":\"BOTTOM\"},\"type\":\"ConnectorPlacement.EquallySpacedRectSide\",\"uuid\":\"136e34fe-1c95-412d-a8c7-b895a3917e8c\"}]},\"type\":\"ConnectorPlacement.EquallySpacedConnector\",\"uuid\":\"b68eec12-5eae-464b-ad0d-c0eefae3b870\"}],\"packageUris\":[\"http://schema.mathworks.com/mf0/Connector/R2020b\"],\"version\":\"1.0\"}"
  Yellow1 : Outport
  Green1 : Outport  Port=2
  Red1 : Outport  Port=3
  Yellow2 : Outport  Port=4
  Green2 : Outport  Port=5
  Red2 : Outport  Port=6
  Yellow3 : Outport  Port=7
  Green3 : Outport  Port=8
  Red3 : Outport  Port=9
  Yellow4 : Outport  Port=10
  Green4 : Outport  Port=11
  Red4 : Outport  Port=12
  Count : Outport  Port=13
  wires:
  Tr_Sys_2/9(Reset) -> Reset_7/1
  Reset_7/1 -> Counter/1
  D Flip-Flop/1 -> AND11/2, AND9/2, AND8/2, AND7/2, AND6/2, AND10/2, AND5/2, AND4/2, AND3/2, AND2/2, AND1/2, AND/2, Tr_Sys_1/1(Counter_ON), Tr_Sys_2/1(Counter_ON), Counter/2
  Tr_Sys_1/1(Yellow_1) -> AND/1
  AND/1 -> Yellow1/1
  Tr_Sys_1/2(Green_1) -> AND1/1
  AND4/1 -> Green2/1
  AND5/1 -> Red2/1
  AND3/1 -> Yellow2/1
  AND2/1 -> Red1/1
  AND1/1 -> Green1/1
  AND6/1 -> Yellow3/1
  Tr_Sys_2/6(Red_4) -> AND11/1
  Tr_Sys_2/5(Green_4) -> AND10/1
  Tr_Sys_2/4(Yellow_4) -> AND9/1
  Tr_Sys_2/3(Red_3) -> AND8/1
  Tr_Sys_2/2(Green_3) -> AND7/1
  Tr_Sys_2/1(Yellow_3) -> AND6/1
  AND11/1 -> Red4/1
  AND10/1 -> Green4/1
  AND9/1 -> Yellow4/1
  AND8/1 -> Red3/1
  AND7/1 -> Green3/1
  Tr_Sys_1/5(Green_2) -> AND4/1
  Tr_Sys_1/6(Red_2) -> AND5/1
  Tr_Sys_1/4(Yellow_2) -> AND3/1
  Tr_Sys_1/3(Red_1) -> AND2/1
  Counter/1 -> Count/1, Tr_Sys_2/2(CountIn), Tr_Sys_1/2(CountIn)
  TrSys_Enb/1 -> D Flip-Flop/1
  Enable/1 -> D Flip-Flop/3
  Clock/1 -> D Flip-Flop/2
  D Flip-Flop/2 -> Terminator/1
  Tr_Sys_1/7(Post1) -> Display/1
  Tr_Sys_2/8(Post4) -> Display1/1
  Tr_Sys_1/8(Post2) -> Display2/1
  Tr_Sys_2/7(Post3) -> Display3/1

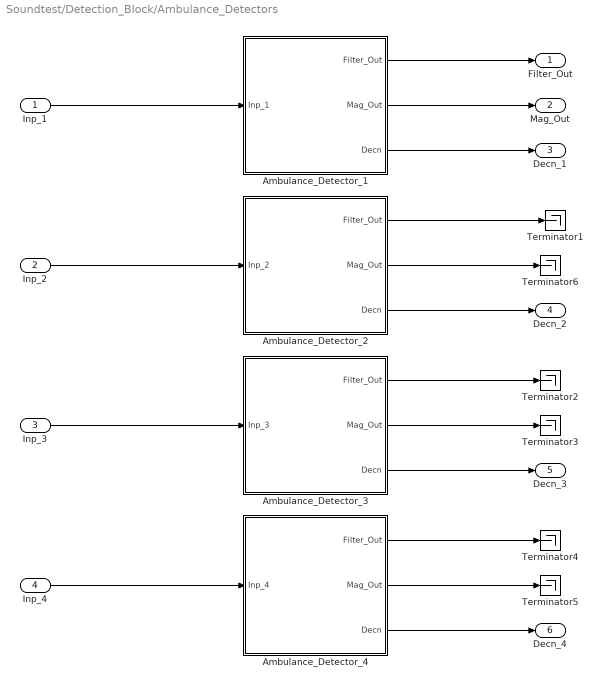
== system Soundtest/Detection_Block/Ambulance_Detectors ==
  Inp_1 : Inport
  Inp_2 : Inport  Port=2
  Inp_3 : Inport  Port=3
  Inp_4 : Inport  Port=4
  Ambulance_Detector_1 : Subsystem
  Ambulance_Detector_2 : Subsystem
  Ambulance_Detector_3 : Subsystem
  Ambulance_Detector_4 : Subsystem
  Terminator{1..6} (6 alike) : Terminator
  Filter_Out : Outport
  Mag_Out : Outport  Port=2
  Decn_1 : Outport  Port=3
  Decn_2 : Outport  Port=4
  Decn_3 : Outport  Port=5
  Decn_4 : Outport  Port=6
  wires:
  Ambulance_Detector_3/2(Mag_Out) -> Terminator3/1
  Ambulance_Detector_2/3(Decn) -> Decn_2/1
  Ambulance_Detector_4/2(Mag_Out) -> Terminator5/1
  Ambulance_Detector_2/2(Mag_Out) -> Terminator6/1
  Ambulance_Detector_2/1(Filter_Out) -> Terminator1/1
  Ambulance_Detector_4/1(Filter_Out) -> Terminator4/1
  Ambulance_Detector_3/3(Decn) -> Decn_3/1
  Ambulance_Detector_3/1(Filter_Out) -> Terminator2/1
  Ambulance_Detector_4/3(Decn) -> Decn_4/1
  Ambulance_Detector_1/2(Mag_Out) -> Mag_Out/1
  Inp_4/1 -> Ambulance_Detector_4/1(Inp_4)
  Ambulance_Detector_1/3(Decn) -> Decn_1/1
  Ambulance_Detector_1/1(Filter_Out) -> Filter_Out/1
  Inp_3/1 -> Ambulance_Detector_3/1(Inp_3)
  Inp_2/1 -> Ambulance_Detector_2/1(Inp_2)
  Inp_1/1 -> Ambulance_Detector_1/1(Inp_1)

== system Soundtest/Detection_Block/Input_Sensors ==
  Sensor_1 : dspvision/From Multimedia File  inputFilename=D:\Technical Softwares\Majot Project\[MONO]Traffic Noise1-320k.mp3  readRange=[1 Inf]  loop=on  numPlays=inf  outputStreams=Audio only  videoDataType=single  audioDataType=double  inheritSampleTime=on  userDefinedSampleTime=1/30  noAudioOutput=off  isIntensityVideo=off  fourcc=RGB  colorVideoFormat=Separate color signals  outputEOF=off  dataOrg=Column-major  audioFrameSize=1  computeAudioFrameSize=off  outSamplingMode=Sample based
  Sensor_2 : dspvision/From Multimedia File  inputFilename=D:\Technical Softwares\Majot Project\[MONO]Traffic Noise1-320k.mp3  readRange=[1 Inf]  loop=on  numPlays=inf  outputStreams=Audio only  videoDataType=single  audioDataType=double  inheritSampleTime=on  userDefinedSampleTime=1/2  noAudioOutput=off  isIntensityVideo=off  fourcc=RGB  colorVideoFormat=Separate color signals  outputEOF=off  dataOrg=Column-major  audioFrameSize=1  computeAudioFrameSize=off  outSamplingMode=Sample based
  Sensor_3 : dspvision/From Multimedia File  inputFilename=D:\Technical Softwares\Majot Project\[MONO]Traffic Sound+Amb Effect-320k.mp3  readRange=[1 Inf]  loop=on  numPlays=inf  outputStreams=Audio only  videoDataType=single  audioDataType=double  inheritSampleTime=on  userDefinedSampleTime=1/2  noAudioOutput=off  isIntensityVideo=off  fourcc=RGB  colorVideoFormat=Separate color signals  outputEOF=off  dataOrg=Column-major  audioFrameSize=1  computeAudioFrameSize=off  outSamplingMode=Sample based
  Sensor_4 : dspvision/From Multimedia File  inputFilename=D:\Technical Softwares\Majot Project\[MONO]Traffic Noise1-320k.mp3  readRange=[1 Inf]  loop=on  numPlays=inf  outputStreams=Audio only  videoDataType=single  audioDataType=double  inheritSampleTime=on  userDefinedSampleTime=1/2  noAudioOutput=off  isIntensityVideo=off  fourcc=RGB  colorVideoFormat=Separate color signals  outputEOF=off  dataOrg=Column-major  audioFrameSize=1  computeAudioFrameSize=off  outSamplingMode=Sample based
  Inp_1 : Outport
  Inp_2 : Outport  Port=2
  Inp_3 : Outport  Port=3
  Inp_4 : Outport  Port=4
  wires:
  Sensor_3/1 -> Inp_3/1
  Sensor_4/1 -> Inp_4/1
  Sensor_2/1 -> Inp_2/1
  Sensor_1/1 -> Inp_1/1

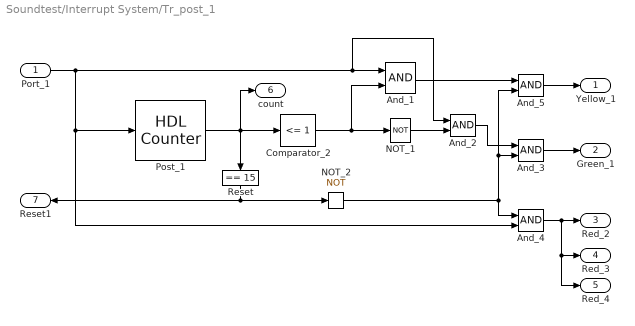
== system Soundtest/Interrupt System/Tr_post_1 ==
  Port_1 : Inport
  And_1 : Logic  AllPortsSameDT=off  OutDataTypeStr=boolean
  And_2 : Logic  AllPortsSameDT=off  OutDataTypeStr=boolean
  And_3 : Logic  IconShape=distinctive  AllPortsSameDT=off  OutDataTypeStr=boolean
  And_4 : Logic  IconShape=distinctive  AllPortsSameDT=off  OutDataTypeStr=boolean
  And_5 : Logic  IconShape=distinctive  AllPortsSameDT=off  OutDataTypeStr=boolean
  Comparator_2 : simulink/Logic and Bit Operations/Compare To Constant  relop=<=  const=1  OutDataTypeStr=boolean
  NOT_1 : Logic  Operator=NOT  IconShape=distinctive  AllPortsSameDT=off  OutDataTypeStr=boolean
  NOT_2 : Logic  Operator=NOT  IconShape=distinctive  AllPortsSameDT=off  OutDataTypeStr=boolean
  Post_1 : hdlsllib/Sources/HDL Counter  CountType=Count limited  CountInit=0  CountStep=1  CountMax=15  CountFromType=Initial value  CountFrom=0  CountResetPort=off  CountLoadPort=off  CountEnbPort=on  CountDirPort=off  CountHitOutputPort=off  CountDataType=Unsigned  CountWordLen=8  CountFracLen=0  CountSampTime=1
  Reset : simulink/Logic and Bit Operations/Compare To Constant  relop===  const=15  OutDataTypeStr=boolean
  Yellow_1 : Outport
  Green_1 : Outport  Port=2
  Red_2 : Outport  Port=3  VectorParamsAs1DForOutWhenUnconnected=off
  Red_3 : Outport  Port=4  VectorParamsAs1DForOutWhenUnconnected=off
  Red_4 : Outport  Port=5  VectorParamsAs1DForOutWhenUnconnected=off
  count : Outport  Port=6
  Reset1 : Outport  Port=7  VectorParamsAs1DForOutWhenUnconnected=off
  wires:
  Port_1/1 -> And_2/1, And_1/1, Post_1/1, And_4/2
  Post_1/1 -> Comparator_2/1, count/1, Reset/1
  Comparator_2/1 -> And_1/2, NOT_1/1
  NOT_1/1 -> And_2/2
  And_2/1 -> And_3/1
  NOT_2/1 -> And_3/2, And_5/2, And_4/1
  And_3/1 -> Green_1/1
  And_4/1 -> Red_4/1, Red_3/1, Red_2/1
  And_1/1 -> And_5/1
  And_5/1 -> Yellow_1/1
  Reset/1 -> Reset1/1, NOT_2/1

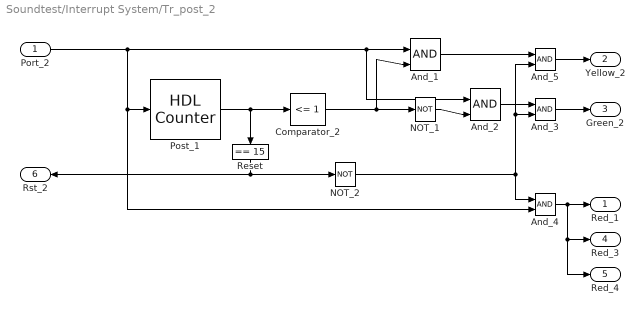
== system Soundtest/Interrupt System/Tr_post_2 ==
  Port_2 : Inport
  And_{1..5} (5 alike) : Logic  IconShape=distinctive  AllPortsSameDT=off  OutDataTypeStr=boolean
  Comparator_2 : simulink/Logic and Bit Operations/Compare To Constant  relop=<=  const=1  OutDataTypeStr=boolean
  NOT_1 : Logic  Operator=NOT  IconShape=distinctive  AllPortsSameDT=off  OutDataTypeStr=boolean
  NOT_2 : Logic  Operator=NOT  IconShape=distinctive  AllPortsSameDT=off  OutDataTypeStr=boolean
  Post_1 : hdlsllib/Sources/HDL Counter  CountType=Count limited  CountInit=0  CountStep=1  CountMax=15  CountFromType=Initial value  CountFrom=0  CountResetPort=off  CountLoadPort=off  CountEnbPort=on  CountDirPort=off  CountHitOutputPort=off  CountDataType=Unsigned  CountWordLen=8  CountFracLen=0  CountSampTime=1
  Reset : simulink/Logic and Bit Operations/Compare To Constant  relop===  const=15  OutDataTypeStr=boolean
  Red_1 : Outport  VectorParamsAs1DForOutWhenUnconnected=off
  Yellow_2 : Outport  Port=2
  Green_2 : Outport  Port=3
  Red_3 : Outport  Port=4  VectorParamsAs1DForOutWhenUnconnected=off
  Red_4 : Outport  Port=5  VectorParamsAs1DForOutWhenUnconnected=off
  Rst_2 : Outport  Port=6
  wires:
  Comparator_2/1 -> NOT_1/1, And_1/2
  Post_1/1 -> Reset/1, Comparator_2/1
  Port_2/1 -> And_2/1, And_1/1, Post_1/1, And_4/2
  NOT_1/1 -> And_2/2
  Reset/1 -> Rst_2/1, NOT_2/1
  And_2/1 -> And_3/1
  NOT_2/1 -> And_4/1, And_5/2, And_3/2
  And_3/1 -> Green_2/1
  And_4/1 -> Red_4/1, Red_3/1, Red_1/1
  And_1/1 -> And_5/1
  And_5/1 -> Yellow_2/1

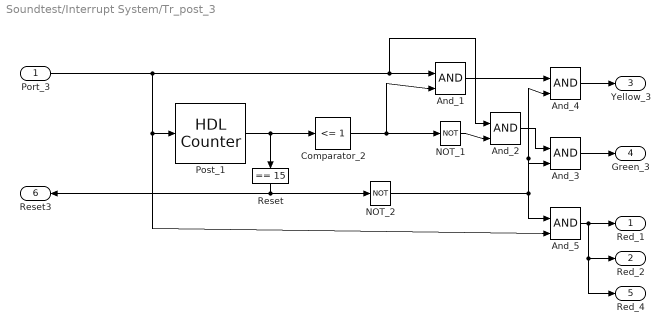
== system Soundtest/Interrupt System/Tr_post_3 ==
  Port_3 : Inport
  And_{1..5} (5 alike) : Logic  IconShape=distinctive  AllPortsSameDT=off  OutDataTypeStr=boolean
  Comparator_2 : simulink/Logic and Bit Operations/Compare To Constant  relop=<=  const=1  OutDataTypeStr=boolean
  NOT_1 : Logic  Operator=NOT  IconShape=distinctive  AllPortsSameDT=off  OutDataTypeStr=boolean
  NOT_2 : Logic  Operator=NOT  IconShape=distinctive  AllPortsSameDT=off  OutDataTypeStr=boolean
  Post_1 : hdlsllib/Sources/HDL Counter  CountType=Count limited  CountInit=0  CountStep=1  CountMax=15  CountFromType=Initial value  CountFrom=0  CountResetPort=off  CountLoadPort=off  CountEnbPort=on  CountDirPort=off  CountHitOutputPort=off  CountDataType=Unsigned  CountWordLen=8  CountFracLen=0  CountSampTime=1
  Reset : simulink/Logic and Bit Operations/Compare To Constant  relop===  const=15  OutDataTypeStr=boolean
  Red_1 : Outport  VectorParamsAs1DForOutWhenUnconnected=off
  Red_2 : Outport  Port=2  VectorParamsAs1DForOutWhenUnconnected=off
  Yellow_3 : Outport  Port=3
  Green_3 : Outport  Port=4
  Red_4 : Outport  Port=5  VectorParamsAs1DForOutWhenUnconnected=off
  Reset3 : Outport  Port=6
  wires:
  Port_3/1 -> And_5/2, Post_1/1, And_2/1, And_1/1
  Post_1/1 -> Comparator_2/1, Reset/1
  Comparator_2/1 -> And_1/2, NOT_1/1
  NOT_1/1 -> And_2/2
  Reset/1 -> NOT_2/1, Reset3/1
  And_1/1 -> And_4/1
  And_4/1 -> Yellow_3/1
  NOT_2/1 -> And_5/1, And_3/2, And_4/2
  And_2/1 -> And_3/1
  And_3/1 -> Green_3/1
  And_5/1 -> Red_1/1, Red_4/1, Red_2/1

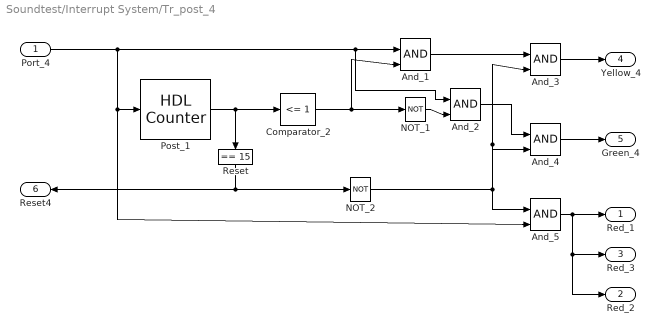
== system Soundtest/Interrupt System/Tr_post_4 ==
  Port_4 : Inport
  And_{1..5} (5 alike) : Logic  IconShape=distinctive  AllPortsSameDT=off  OutDataTypeStr=boolean
  Comparator_2 : simulink/Logic and Bit Operations/Compare To Constant  relop=<=  const=1  OutDataTypeStr=boolean
  NOT_1 : Logic  Operator=NOT  IconShape=distinctive  AllPortsSameDT=off  OutDataTypeStr=boolean
  NOT_2 : Logic  Operator=NOT  IconShape=distinctive  AllPortsSameDT=off  OutDataTypeStr=boolean
  Post_1 : hdlsllib/Sources/HDL Counter  CountType=Count limited  CountInit=0  CountStep=1  CountMax=15  CountFromType=Initial value  CountFrom=0  CountResetPort=off  CountLoadPort=off  CountEnbPort=on  CountDirPort=off  CountHitOutputPort=off  CountDataType=Unsigned  CountWordLen=8  CountFracLen=0  CountSampTime=1
  Reset : simulink/Logic and Bit Operations/Compare To Constant  relop===  const=15  OutDataTypeStr=boolean
  Red_1 : Outport  VectorParamsAs1DForOutWhenUnconnected=off
  Red_2 : Outport  Port=2  VectorParamsAs1DForOutWhenUnconnected=off
  Red_3 : Outport  Port=3  VectorParamsAs1DForOutWhenUnconnected=off
  Yellow_4 : Outport  Port=4
  Green_4 : Outport  Port=5
  Reset4 : Outport  Port=6
  wires:
  Comparator_2/1 -> NOT_1/1, And_1/2
  Post_1/1 -> Reset/1, Comparator_2/1
  Port_4/1 -> And_1/1, And_2/1, Post_1/1, And_5/2
  NOT_1/1 -> And_2/2
  Reset/1 -> NOT_2/1, Reset4/1
  NOT_2/1 -> And_5/1, And_3/2, And_4/2
  And_5/1 -> Red_2/1, Red_3/1, Red_1/1
  And_4/1 -> Green_4/1
  And_3/1 -> Yellow_4/1
  And_2/1 -> And_4/1
  And_1/1 -> And_3/1

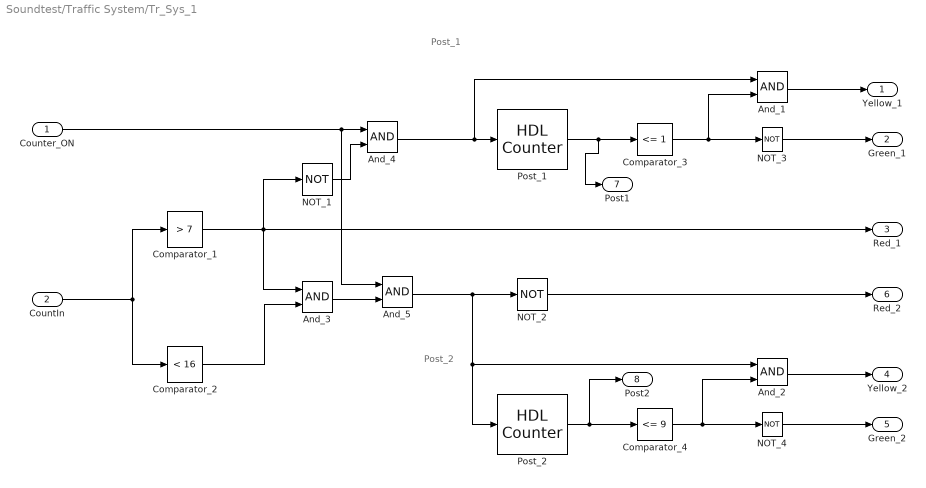
== system Soundtest/Traffic System/Tr_Sys_1 ==
  note: Post_2
  note: Post_1
  Counter_ON : Inport
  CountIn : Inport  Port=2
  And_{1..5} (5 alike) : Logic  AllPortsSameDT=off  OutDataTypeStr=boolean
  Comparator_1 : simulink/Logic and Bit Operations/Compare To Constant  relop=>  const=7  OutDataTypeStr=boolean
  Comparator_2 : simulink/Logic and Bit Operations/Compare To Constant  relop=<  const=16  OutDataTypeStr=boolean
  Comparator_3 : simulink/Logic and Bit Operations/Compare To Constant  relop=<=  const=1  OutDataTypeStr=boolean
  Comparator_4 : simulink/Logic and Bit Operations/Compare To Constant  relop=<=  const=9  OutDataTypeStr=boolean
  NOT_{1..4} (4 alike) : Logic  Operator=NOT  IconShape=distinctive  AllPortsSameDT=off  OutDataTypeStr=boolean
  Post_1 : hdlsllib/Sources/HDL Counter  CountType=Count limited  CountInit=0  CountStep=1  CountMax=7  CountFromType=Initial value  CountFrom=0  CountResetPort=off  CountLoadPort=off  CountEnbPort=on  CountDirPort=off  CountHitOutputPort=off  CountDataType=Unsigned  CountWordLen=8  CountFracLen=0  CountSampTime=1
  Post_2 : hdlsllib/Sources/HDL Counter  CountType=Count limited  CountInit=8  CountStep=1  CountMax=15  CountFromType=Initial value  CountFrom=8  CountResetPort=off  CountLoadPort=off  CountEnbPort=on  CountDirPort=off  CountHitOutputPort=off  CountDataType=Unsigned  CountWordLen=8  CountFracLen=0  CountSampTime=1
  Yellow_1 : Outport
  Green_1 : Outport  Port=2
  Red_1 : Outport  Port=3
  Yellow_2 : Outport  Port=4
  Green_2 : Outport  Port=5
  Red_2 : Outport  Port=6
  Post1 : Outport  Port=7
  Post2 : Outport  Port=8
  wires:
  CountIn/1 -> Comparator_2/1, Comparator_1/1
  Post_1/1 -> Post1/1, Comparator_3/1
  NOT_2/1 -> Red_2/1
  Post_2/1 -> Post2/1, Comparator_4/1
  NOT_4/1 -> Green_2/1
  Comparator_4/1 -> And_2/2, NOT_4/1
  Comparator_3/1 -> NOT_3/1, And_1/2
  And_5/1 -> Post_2/1, And_2/1, NOT_2/1
  NOT_3/1 -> Green_1/1
  And_1/1 -> Yellow_1/1
  And_2/1 -> Yellow_2/1
  Comparator_1/1 -> Red_1/1, And_3/1, NOT_1/1
  Comparator_2/1 -> And_3/2
  And_4/1 -> And_1/1, Post_1/1
  NOT_1/1 -> And_4/2
  Counter_ON/1 -> And_5/1, And_4/1
  And_3/1 -> And_5/2

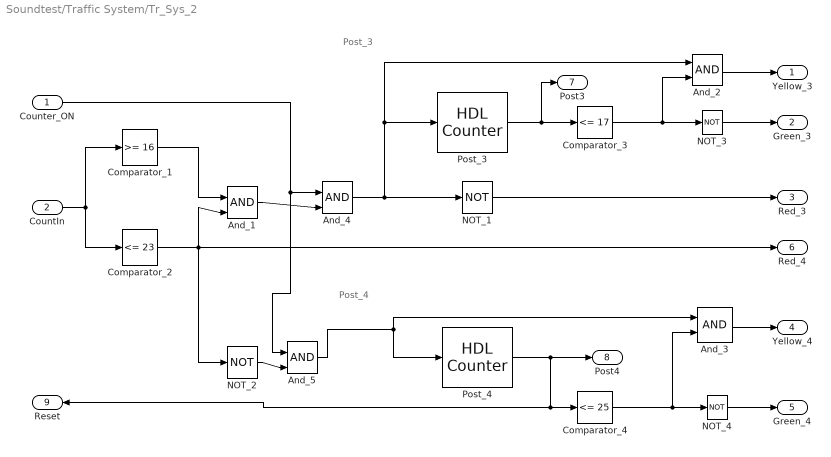
== system Soundtest/Traffic System/Tr_Sys_2 ==
  note: Post_4
  note: Post_3
  Counter_ON : Inport
  CountIn : Inport  Port=2
  And_1 : Logic  IconShape=distinctive  AllPortsSameDT=off  OutDataTypeStr=boolean
  And_2 : Logic  AllPortsSameDT=off  OutDataTypeStr=boolean
  And_3 : Logic  AllPortsSameDT=off  OutDataTypeStr=boolean
  And_4 : Logic  IconShape=distinctive  AllPortsSameDT=off  OutDataTypeStr=boolean
  And_5 : Logic  IconShape=distinctive  AllPortsSameDT=off  OutDataTypeStr=boolean
  Comparator_1 : simulink/Logic and Bit Operations/Compare To Constant  relop=>=  const=16  OutDataTypeStr=boolean
  Comparator_2 : simulink/Logic and Bit Operations/Compare To Constant  relop=<=  const=23  OutDataTypeStr=boolean
  Comparator_3 : simulink/Logic and Bit Operations/Compare To Constant  relop=<=  const=17  OutDataTypeStr=boolean
  Comparator_4 : simulink/Logic and Bit Operations/Compare To Constant  relop=<=  const=25  OutDataTypeStr=boolean
  NOT_{1..4} (4 alike) : Logic  Operator=NOT  IconShape=distinctive  AllPortsSameDT=off  OutDataTypeStr=boolean
  Post_3 : hdlsllib/Sources/HDL Counter  CountType=Count limited  CountInit=16  CountStep=1  CountMax=23  CountFromType=Initial value  CountFrom=16  CountResetPort=off  CountLoadPort=off  CountEnbPort=on  CountDirPort=off  CountHitOutputPort=off  CountDataType=Unsigned  CountWordLen=8  CountFracLen=0  CountSampTime=1
  Post_4 : hdlsllib/Sources/HDL Counter  CountType=Count limited  CountInit=24  CountStep=1  CountMax=31  CountFromType=Initial value  CountFrom=24  CountResetPort=off  CountLoadPort=off  CountEnbPort=on  CountDirPort=off  CountHitOutputPort=off  CountDataType=Unsigned  CountWordLen=8  CountFracLen=0  CountSampTime=1
  Yellow_3 : Outport
  Green_3 : Outport  Port=2
  Red_3 : Outport  Port=3
  Yellow_4 : Outport  Port=4
  Green_4 : Outport  Port=5
  Red_4 : Outport  Port=6
  Post3 : Outport  Port=7
  Post4 : Outport  Port=8
  Reset : Outport  Port=9
  wires:
  Comparator_2/1 -> And_1/2, NOT_2/1, Red_4/1
  NOT_3/1 -> Green_3/1
  And_3/1 -> Yellow_4/1
  Comparator_4/1 -> And_3/2, NOT_4/1
  And_2/1 -> Yellow_3/1
  Comparator_3/1 -> NOT_3/1, And_2/2
  Post_3/1 -> Post3/1, Comparator_3/1
  CountIn/1 -> Comparator_1/1, Comparator_2/1
  NOT_4/1 -> Green_4/1
  Comparator_1/1 -> And_1/1
  And_4/1 -> And_2/1, Post_3/1, NOT_1/1
  NOT_1/1 -> Red_3/1
  And_5/1 -> Post_4/1, And_3/1
  And_1/1 -> And_4/2
  Counter_ON/1 -> And_5/1, And_4/1
  NOT_2/1 -> And_5/2
  Post_4/1 -> Reset/1, Comparator_4/1, Post4/1

== system Soundtest/Detection_Block/Ambulance_Detectors/Ambulance_Detector_1 ==
  Inp_1 : Inport
  Bandpass_Filter : Subsystem  DialogController=fdesignblkfcn  InitFcn=fdesignblkfcn(gcbh, {'InitFcn'});  mask(Bandpass Filter){}
      mask help: Design a bandpass filter
      settings: CopyFcn=fdesignblkfcn(gcbh, {'CopyFcn'});
      mask Help: helpview(mapfilelocation('dsp'), 'dspbandpassfilter');
      mask Display: disp('Bandpass');
  Comparator : simulink/Logic and Bit Operations/Compare To Constant  relop=>=  const=0.8  OutDataTypeStr=boolean  ZeroCross=off
  Complex _to_Magnitude : ComplexToMagnitudeAngle  Output=Magnitude
  Gain : Gain  Gain=2
  Rate Transition : RateTransition  OutPortSampleTime=1
  Filter_Out : Outport
  Mag_Out : Outport  Port=2
  Decn : Outport  Port=3
  wires:
  Complex _to_Magnitude/1 -> Mag_Out/1, Comparator/1
  Inp_1/1 -> Bandpass_Filter/1(In)
  Comparator/1 -> Decn/1
  Rate Transition/1 -> Gain/1
  Bandpass_Filter/1(Out) -> Rate Transition/1
  Gain/1 -> Filter_Out/1, Complex _to_Magnitude/1

== system Soundtest/Detection_Block/Ambulance_Detectors/Ambulance_Detector_2 ==
  Inp_2 : Inport
  Bandpass_Filter : Subsystem  DialogController=fdesignblkfcn  InitFcn=fdesignblkfcn(gcbh, {'InitFcn'});  mask(Bandpass Filter){}
      mask help: Design a bandpass filter
      settings: CopyFcn=fdesignblkfcn(gcbh, {'CopyFcn'});
      mask Help: helpview(mapfilelocation('dsp'), 'dspbandpassfilter');
      mask Display: disp('Bandpass');
  Comparator : simulink/Logic and Bit Operations/Compare To Constant  relop=>=  const=0.8  OutDataTypeStr=boolean  ZeroCross=off
  Complex _to_Magnitude : ComplexToMagnitudeAngle  Output=Magnitude
  Gain : Gain  Gain=2
  Rate Transition : RateTransition  OutPortSampleTime=1
  Filter_Out : Outport
  Mag_Out : Outport  Port=2
  Decn : Outport  Port=3
  wires:
  Inp_2/1 -> Bandpass_Filter/1(In)
  Comparator/1 -> Decn/1
  Complex _to_Magnitude/1 -> Comparator/1, Mag_Out/1
  Gain/1 -> Complex _to_Magnitude/1, Filter_Out/1
  Rate Transition/1 -> Gain/1
  Bandpass_Filter/1(Out) -> Rate Transition/1

== system Soundtest/Detection_Block/Ambulance_Detectors/Ambulance_Detector_3 ==
  Inp_3 : Inport
  Bandpass_Filter : Subsystem  DialogController=fdesignblkfcn  InitFcn=fdesignblkfcn(gcbh, {'InitFcn'});  mask(Bandpass Filter){}
      mask help: Design a bandpass filter
      settings: CopyFcn=fdesignblkfcn(gcbh, {'CopyFcn'});
      mask Help: helpview(mapfilelocation('dsp'), 'dspbandpassfilter');
      mask Display: disp('Bandpass');
  Comparator : simulink/Logic and Bit Operations/Compare To Constant  relop=>=  const=0.8  OutDataTypeStr=boolean  ZeroCross=off
  Complex _to_Magnitude : ComplexToMagnitudeAngle  Output=Magnitude
  Gain : Gain  Gain=2
  Rate Transition : RateTransition  OutPortSampleTime=1
  Filter_Out : Outport
  Mag_Out : Outport  Port=2
  Decn : Outport  Port=3
  wires:
  Gain/1 -> Filter_Out/1, Complex _to_Magnitude/1
  Complex _to_Magnitude/1 -> Mag_Out/1, Comparator/1
  Comparator/1 -> Decn/1
  Inp_3/1 -> Bandpass_Filter/1(In)
  Rate Transition/1 -> Gain/1
  Bandpass_Filter/1(Out) -> Rate Transition/1

== system Soundtest/Detection_Block/Ambulance_Detectors/Ambulance_Detector_4 ==
  Inp_4 : Inport
  Bandpass_Filter : Subsystem  DialogController=fdesignblkfcn  InitFcn=fdesignblkfcn(gcbh, {'InitFcn'});  mask(Bandpass Filter){}
      mask help: Design a bandpass filter
      settings: CopyFcn=fdesignblkfcn(gcbh, {'CopyFcn'});
      mask Help: helpview(mapfilelocation('dsp'), 'dspbandpassfilter');
      mask Display: disp('Bandpass');
  Comparator : simulink/Logic and Bit Operations/Compare To Constant  relop=>=  const=0.8  OutDataTypeStr=boolean  ZeroCross=off
  Complex _to_Magnitude : ComplexToMagnitudeAngle  Output=Magnitude
  Filter_Out : Outport
  Mag_Out : Outport  Port=2
  Decn : Outport  Port=3
  wires:
  Inp_4/1 -> Bandpass_Filter/1(In)
  Comparator/1 -> Decn/1
  Complex _to_Magnitude/1 -> Comparator/1, Mag_Out/1
  Bandpass_Filter/1(Out) -> Complex _to_Magnitude/1, Filter_Out/1
